simulink model "main_bsm_sl"  (R2023b)
settings: Solver=VariableStepAuto  StartTime=0.0  StopTime=10.0  RelTol=1e-3
undefined symbols (not defined in the file or in its folder): bsm
settings Model: Creator=tard  LastModifiedBy=tard

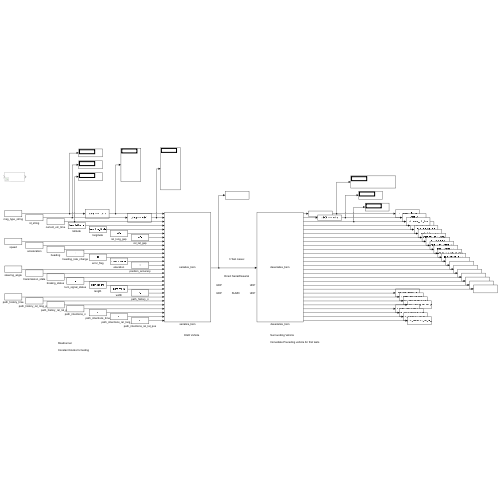
[thumbnail: Simulink's stored preview of the top-level diagram]
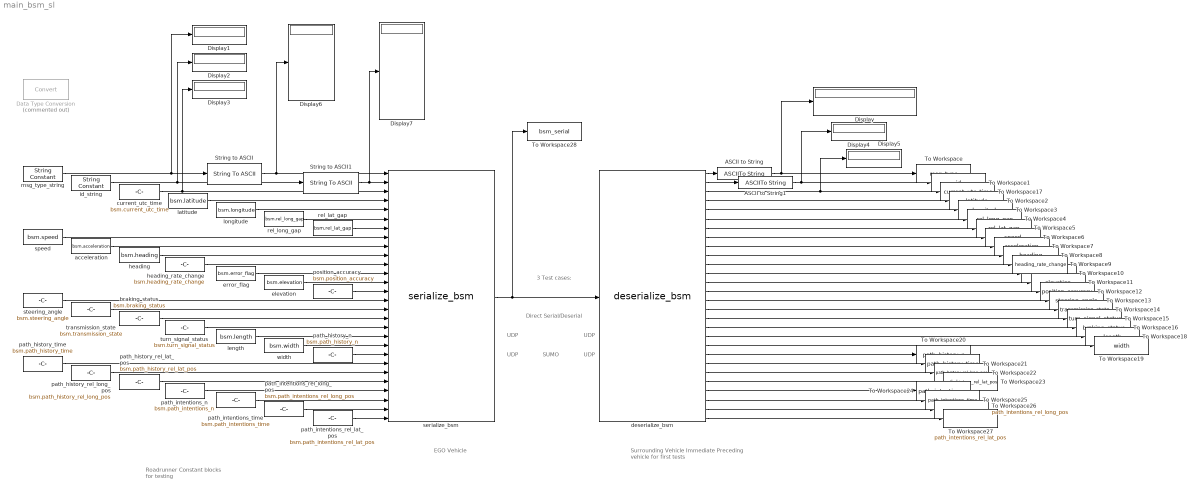
== system main_bsm_sl ==
  note: Direct Serial/Deserial
  note: 3 Test cases:
  note: Surrounding Vehicle
      |
      | Immediate Preceding vehicle for first tests
  note: EGO Vehicle
  note: SUMO
  note: UDP
  note: Roadrunner
      |
      | Constant blocks for testing
  note: UDP
  note: UDP
  note: UDP
  ASCII to String : ASCIIToString
  ASCII to String1 : ASCIIToString
  Data Type Conversion : DataTypeConversion  Commented=on  SaturateOnIntegerOverflow=off  RndMeth=Floor
  Display{,1..7} (8 alike) : Display
  String to ASCII : StringToASCII
  String to ASCII1 : StringToASCII
  To Workspace : ToWorkspace  VariableName=msg_type  SaveFormat=Timeseries  SampleTime=-1
  To Workspace1 : ToWorkspace  VariableName=id  SaveFormat=Timeseries  SampleTime=-1
  To Workspace10 : ToWorkspace  VariableName=error_flag  SaveFormat=Timeseries  SampleTime=-1
  To Workspace11 : ToWorkspace  VariableName=elevation  SaveFormat=Timeseries  SampleTime=-1
  To Workspace12 : ToWorkspace  VariableName=position_accuracy  SaveFormat=Timeseries  SampleTime=-1
  To Workspace13 : ToWorkspace  VariableName=steering_angle  SaveFormat=Timeseries  SampleTime=-1
  To Workspace14 : ToWorkspace  VariableName=transmission_state  SaveFormat=Timeseries  SampleTime=-1
  To Workspace15 : ToWorkspace  VariableName=turn_signal_status  SaveFormat=Timeseries  SampleTime=-1
  To Workspace16 : ToWorkspace  VariableName=braking_status  SaveFormat=Timeseries  SampleTime=-1
  To Workspace17 : ToWorkspace  VariableName=current_utc_time  SaveFormat=Timeseries  SampleTime=-1
  To Workspace18 : ToWorkspace  VariableName=length  SaveFormat=Timeseries  SampleTime=-1
  To Workspace19 : ToWorkspace  VariableName=width  SaveFormat=Timeseries  SampleTime=-1
  To Workspace2 : ToWorkspace  VariableName=latitude  SaveFormat=Timeseries  SampleTime=-1
  To Workspace20 : ToWorkspace  VariableName=path_history_n  SaveFormat=Timeseries  SampleTime=-1
  To Workspace21 : ToWorkspace  VariableName=path_history_time  SaveFormat=Timeseries  SampleTime=-1
  To Workspace22 : ToWorkspace  VariableName=path_history_rel_long_pos  SaveFormat=Timeseries  SampleTime=-1
  To Workspace23 : ToWorkspace  VariableName=path_history_rel_lat_pos  SaveFormat=Timeseries  SampleTime=-1
  To Workspace24 : ToWorkspace  VariableName=path_intentions_n  SaveFormat=Timeseries  SampleTime=-1
  To Workspace25 : ToWorkspace  VariableName=path_intentions_time  SaveFormat=Timeseries  SampleTime=-1
  To Workspace26 : ToWorkspace  VariableName=path_intentions_rel_long_pos  SaveFormat=Timeseries  SampleTime=-1
  To Workspace27 : ToWorkspace  VariableName=path_intentions_rel_lat_pos  SaveFormat=Timeseries  SampleTime=-1
  To Workspace28 : ToWorkspace  VariableName=bsm_serial  SaveFormat=Timeseries  SampleTime=-1
  To Workspace3 : ToWorkspace  VariableName=longitude  SaveFormat=Timeseries  SampleTime=-1
  To Workspace4 : ToWorkspace  VariableName=rel_long_gap  SaveFormat=Timeseries  SampleTime=-1
  To Workspace5 : ToWorkspace  VariableName=rel_lat_gap  SaveFormat=Timeseries  SampleTime=-1
  To Workspace6 : ToWorkspace  VariableName=speed  SaveFormat=Timeseries  SampleTime=-1
  To Workspace7 : ToWorkspace  VariableName=acceleration  SaveFormat=Timeseries  SampleTime=-1
  To Workspace8 : ToWorkspace  VariableName=heading  SaveFormat=Timeseries  SampleTime=-1
  To Workspace9 : ToWorkspace  VariableName=heading_rate_change  SaveFormat=Timeseries  SampleTime=-1
  acceleration : Constant  Value=bsm.acceleration
  braking_status : Constant  Value=bsm.braking_status
  current_utc_time : Constant  Value=bsm.current_utc_time
  deserialize_bsm : S-Function  FunctionName=deserialize_bsm  SFunctionDeploymentMode=off  EnableBusSupport=off
  elevation : Constant  Value=bsm.elevation
  error_flag : Constant  Value=bsm.error_flag
  heading : Constant  Value=bsm.heading
  heading_rate_change : Constant  Value=bsm.heading_rate_change
  id_string : StringConstant  String=bsm.id
  latitude : Constant  Value=bsm.latitude
  length : Constant  Value=bsm.length
  longitude : Constant  Value=bsm.longitude
  msg_type_string : StringConstant  String=bsm.msg_type
  path_history_n : Constant  Value=bsm.path_history_n
  path_history_rel_lat_pos : Constant  Value=bsm.path_history_rel_lat_pos
  path_history_rel_long_pos : Constant  Value=bsm.path_history_rel_long_pos
  path_history_time : Constant  Value=bsm.path_history_time
  path_intentions_n : Constant  Value=bsm.path_intentions_n
  path_intentions_rel_lat_pos : Constant  Value=bsm.path_intentions_rel_lat_pos
  path_intentions_rel_long_pos : Constant  Value=bsm.path_intentions_rel_long_pos
  path_intentions_time : Constant  Value=bsm.path_intentions_time
  position_accuracy : Constant  Value=bsm.position_accuracy
  rel_lat_gap : Constant  Value=bsm.rel_lat_gap
  rel_long_gap : Constant  Value=bsm.rel_long_gap
  serialize_bsm : S-Function  FunctionName=serialize_bsm  SFunctionDeploymentMode=off  EnableBusSupport=off
  speed : Constant  Value=bsm.speed
  steering_angle : Constant  Value=bsm.steering_angle
  transmission_state : Constant  Value=bsm.transmission_state
  turn_signal_status : Constant  Value=bsm.turn_signal_status
  width : Constant  Value=bsm.width
  wires:
  ASCII to String/1 -> Display/1, To Workspace/1
  deserialize_bsm/2 -> ASCII to String1/1
  deserialize_bsm/3 -> To Workspace17/1, Display5/1
  deserialize_bsm/18 -> To Workspace16/1
  deserialize_bsm/19 -> To Workspace18/1
  deserialize_bsm/20 -> To Workspace19/1
  deserialize_bsm/21 -> To Workspace20/1
  deserialize_bsm/22 -> To Workspace21/1
  deserialize_bsm/23 -> To Workspace22/1
  deserialize_bsm/24 -> To Workspace23/1
  deserialize_bsm/25 -> To Workspace24/1
  deserialize_bsm/26 -> To Workspace25/1
  deserialize_bsm/27 -> To Workspace26/1
  deserialize_bsm/28 -> To Workspace27/1
  serialize_bsm/1 -> deserialize_bsm/1, To Workspace28/1
  latitude/1 -> serialize_bsm/4
  current_utc_time/1 -> serialize_bsm/3, Display3/1
  longitude/1 -> serialize_bsm/5
  speed/1 -> serialize_bsm/8
  acceleration/1 -> serialize_bsm/9
  heading/1 -> serialize_bsm/10
  heading_rate_change/1 -> serialize_bsm/11
  error_flag/1 -> serialize_bsm/12
  elevation/1 -> serialize_bsm/13
  position_accuracy/1 -> serialize_bsm/14
  steering_angle/1 -> serialize_bsm/15
  transmission_state/1 -> serialize_bsm/16
  braking_status/1 -> serialize_bsm/17
  turn_signal_status/1 -> serialize_bsm/18
  length/1 -> serialize_bsm/19
  width/1 -> serialize_bsm/20
  path_history_n/1 -> serialize_bsm/21
  path_history_time/1 -> serialize_bsm/22
  path_history_rel_long_pos/1 -> serialize_bsm/23
  path_history_rel_lat_pos/1 -> serialize_bsm/24
  path_intentions_n/1 -> serialize_bsm/25
  path_intentions_time/1 -> serialize_bsm/26
  path_intentions_rel_long_pos/1 -> serialize_bsm/27
  path_intentions_rel_lat_pos/1 -> serialize_bsm/28
  id_string/1 -> String to ASCII1/1, Display2/1
  msg_type_string/1 -> String to ASCII/1, Display1/1
  rel_long_gap/1 -> serialize_bsm/6
  rel_lat_gap/1 -> serialize_bsm/7
  String to ASCII/1 -> Display6/1, serialize_bsm/1
  String to ASCII1/1 -> serialize_bsm/2, Display7/1
  deserialize_bsm/1 -> ASCII to String/1
  ASCII to String1/1 -> Display4/1, To Workspace1/1
  deserialize_bsm/4 -> To Workspace2/1
  deserialize_bsm/5 -> To Workspace3/1
  deserialize_bsm/6 -> To Workspace4/1
  deserialize_bsm/7 -> To Workspace5/1
  deserialize_bsm/8 -> To Workspace6/1
  deserialize_bsm/9 -> To Workspace7/1
  deserialize_bsm/10 -> To Workspace8/1
  deserialize_bsm/11 -> To Workspace9/1
  deserialize_bsm/12 -> To Workspace10/1
  deserialize_bsm/13 -> To Workspace11/1
  deserialize_bsm/14 -> To Workspace12/1
  deserialize_bsm/15 -> To Workspace13/1
  deserialize_bsm/16 -> To Workspace14/1
  deserialize_bsm/17 -> To Workspace15/1
